simulink model "WhiteBlancing_using_Intensity_Values_of_full_Image"  (R2016a)
settings: Solver=VariableStepAuto  StartTime=0.0  StopTime=10.0  RelTol=1e-3
libraries: visionsinks x2, visionsources x1
settings Model: Creator=YASARA  LastModifiedBy=YASARA

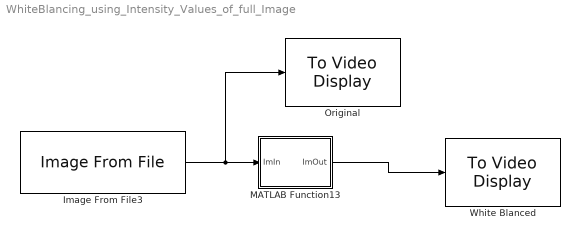
== system WhiteBlancing_using_Intensity_Values_of_full_Image ==
  Image From File3 : visionsources/Image From File  Tag=vipblks_nd  FileName=C:\Users\YASARA\Desktop\FRY_Docu\tea\teaxb.jpg  imagePorts=One multidimensional signal  Ts=1  ImageDataType=uint8  Signed=on  WordLength=16  sdImageDataType=uint(8)  FractionLengthMode=User-defined  FractionLength=15  OutPortLabels=R|G|B
  MATLAB Function13 : MATLAB Function  TreatAsAtomicUnit=on
  Original : visionsinks/To Video Display  windowSizeMode=Normal  openAtMdlStart=on  fullScreen=off  videoWindowX=43  videoWindowY=31  saveWindowSize=off  videoWindowWidth=915  videoWindowHeight=741  inputColorFormat=RGB  inputType=Obsolete  imagePorts=One multidimensional signal  OutputDevice=On-screen video monitor  dataOrg=Column-major  isWindowOpen=off
  White Blanced : visionsinks/To Video Display  windowSizeMode=Normal  openAtMdlStart=on  fullScreen=off  videoWindowX=43  videoWindowY=31  saveWindowSize=off  videoWindowWidth=915  videoWindowHeight=741  inputColorFormat=RGB  inputType=Obsolete  imagePorts=One multidimensional signal  OutputDevice=On-screen video monitor  dataOrg=Column-major  isWindowOpen=off
  wires:
  Image From File3/1 -> Original/1, MATLAB Function13/1(ImIn)
  MATLAB Function13/1(ImOut) -> White Blanced/1

== matlab function WhiteBlancing_using_Intensity_Values_of_full_Image/MATLAB Function13 ==
  data: ImIn input; ImOut output
function ImOut = fcn(ImIn)
ImOut=ImIn;
grayImage = rgb2gray(ImIn);
redChannel = ImIn(:, :, 1);
greenChannel = ImIn(:, :, 2);
blueChannel = ImIn(:, :, 3);
meanR = mean2(redChannel);
meanG = mean2(greenChannel);
meanB = mean2(blueChannel);
meanGray = mean2(grayImage);
redChannel = uint8(double(redChannel) * meanGray / meanR);
greenChannel = uint8(double(greenChannel) * meanGray / meanG);
blueChannel = uint8(double(blueChannel) * meanGray / meanB);
ImOut = cat(3, redChannel, greenChannel, blueChannel);
